simulink model "Bintang_Latihan_Spring_Damper"  (R2023a)
settings: Solver=VariableStepAuto  StartTime=0.0  StopTime=100  RelTol=1e-3
values from neighbouring files (symbols this model uses):
  c = 6    [m_File2.mat]
  dxdt_init = 0    [m_File2.mat]
  k = 2    [m_File2.mat]
  m = 25    [m_File2.mat]
  t_step_F = 75    [m_File2.mat]
  x_init = 5    [m_File2.mat]
settings Model: Creator=Lenovo  LastModifiedBy=Lenovo

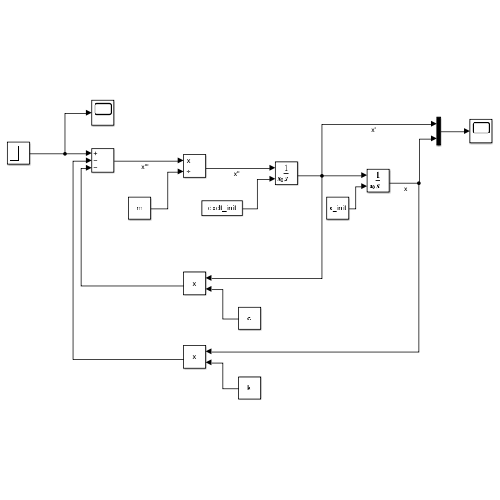
[thumbnail: Simulink's stored preview of the top-level diagram]
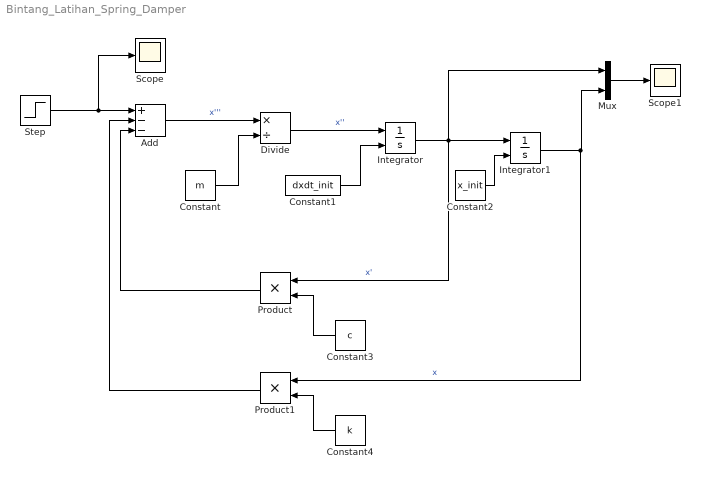
== system Bintang_Latihan_Spring_Damper ==
  Add : Sum  Inputs=+--
  Constant : Constant  Value=m
  Constant1 : Constant  Value=dxdt_init
  Constant2 : Constant  Value=x_init
  Constant3 : Constant  Value=c
  Constant4 : Constant  Value=k
  Divide : Product  Inputs=*/
  Integrator : Integrator  InitialConditionSource=external
  Integrator1 : Integrator  InitialConditionSource=external
  Mux : Mux  Inputs=2
  Product : Product
  Product1 : Product
  Scope : Scope
  Scope1 : Scope
  Step : Step  Time=t_step_F  After=c  SampleTime=0
  wires:
  Integrator/1 -> Mux/1, Product/1, Integrator1/1  "x'"
  Constant4/1 -> Product1/2
  Product1/1 -> Add/2
  Add/1 -> Divide/1  "x'''"
  Integrator1/1 -> Product1/1, Mux/2  "x"
  Divide/1 -> Integrator/1  "x''"
  Constant2/1 -> Integrator1/2
  Constant3/1 -> Product/2
  Product/1 -> Add/3
  Mux/1 -> Scope1/1
  Step/1 -> Scope/1, Add/1
  Constant1/1 -> Integrator/2
  Constant/1 -> Divide/2
